simulink model "Comparative"  (R2022a)
settings: Solver=ode45  StartTime=0.0  StopTime=10  MaxStep=0.1  RelTol=1e-3  EnableMultiTasking=on
values from neighbouring files (symbols this model uses):
  fi0 = 30    [parameters.m]
  kd = 0.1537    [parameters.m]
  ki = 768.3330    (= 768.333)    [parameters.m]
  kp = 23.0500    (= 23.05)    [parameters.m]
  kp_angle = 6    [parameters.m]
  v0 = 0    [parameters.m]
libraries: fuzblock x1
settings Model: Creator=JM  LastModifiedBy=josem
settings SolverCC: AlgebraicLoopSolver=TrustRegion
settings DataIOCC: LimitDataPoints=on  SaveFormat=Array  ReturnWorkspaceOutputs=off
settings OptimizationCC: LifeSpan=inf
settings DebuggingCC: UnconnectedInputMsg=warning  UnconnectedOutputMsg=warning  UnconnectedLineMsg=warning  SFUnexpectedBacktrackingDiag=warning  SFNoUnconditionalDefaultTransitionDiag=warning  SFExecutionAtInitializationDiag=none  SFMachineParentedDataDiag=warning  ArithmeticOperatorsInVariantConditions=warning
settings HardwareCC: ProdBitPerPointer=32  ProdBitPerSizeT=32  ProdBitPerPtrDiffT=32  ProdLargestAtomicFloat=None  ProdIntDivRoundTo=Undefined  ProdEndianess=Unspecified  ProdWordSize=32  ProdHWDeviceType=32-bit Generic
settings ModelReferenceCC: PropagateSignalLabelsOutOfModel=off
settings SFSimCC: SimUseLocalCustomCode=off  CustomCodeUndefinedFunction=UseInterfaceOnly
settings RTWCC: RTWUseLocalCustomCode=off
settings CodeAppCC: StateflowObjectComments=on
settings GRTTargetCC: TargetLangStandard=C89/C90 (ANSI)
settings ConfigComp: CovMetricSettings=dw  CovSaveCumulativeToWorkspaceVar=on  CovSaveSingleToWorkspaceVar=on  CovExternalEMLEnable=off

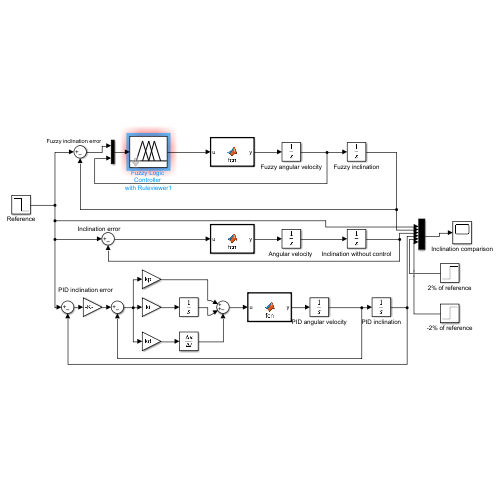
[thumbnail: Simulink's stored preview of the top-level diagram]
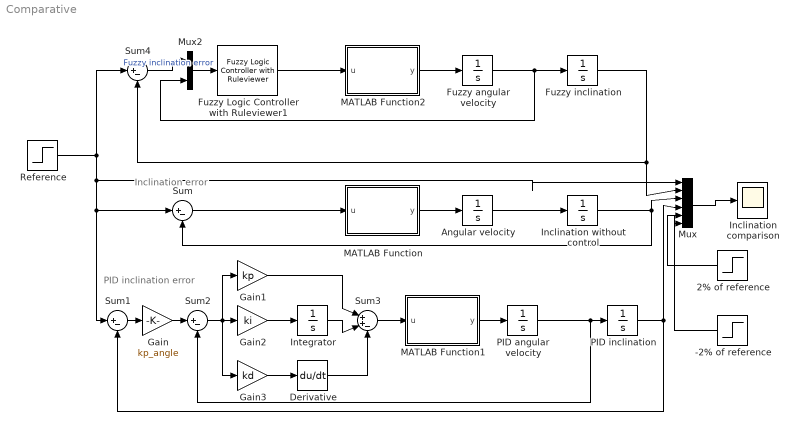
== system Comparative ==
  note: PID inclination error
  note: Inclination error
  -2% of reference : Step  Time=0  Before=-fi0*0.02  After=-fi0*0.02  SampleTime=0
  2% of reference : Step  Time=0  Before=fi0*0.02  After=fi0*0.02  SampleTime=0
  "Angular velocity " : Integrator  InitialCondition=v0
  Derivative : Derivative
  Fuzzy Logic Controller with Ruleviewer1 : fuzblock/Fuzzy Logic  Controller  with Ruleviewer  fismatrix=ControlFuzzy  Ts=0.1
  Fuzzy angular velocity : Integrator  InitialCondition=v0
  Fuzzy inclination : Integrator  InitialCondition=fi0
  Gain : Gain  Gain=kp_angle
  Gain1 : Gain  Gain=kp
  Gain2 : Gain  Gain=ki
  Gain3 : Gain  Gain=kd
  Inclination comparison : Scope
  Inclination without control : Integrator  InitialCondition=fi0
  Integrator : Integrator
  MATLAB Function : MATLAB Function  TreatAsAtomicUnit=on
  MATLAB Function1 : MATLAB Function  TreatAsAtomicUnit=on
  MATLAB Function2 : MATLAB Function  TreatAsAtomicUnit=on
  Mux : Mux  Inputs=6
  Mux2 : Mux  Inputs=2
  PID angular velocity : Integrator  InitialCondition=v0
  PID inclination : Integrator  InitialCondition=fi0
  Reference : Step  Before=fi0  After=0  SampleTime=0
  Sum{,1..2,4} (4 alike) : Sum  Inputs=|+-
  Sum3 : Sum  Inputs=|++-
  wires:
  "Angular velocity "/1 -> Inclination without control/1
  MATLAB Function/1(y) -> "Angular velocity "/1
  Inclination without control/1 -> Sum/2, Mux/3
  Mux/1 -> Inclination comparison/1
  Sum/1 -> MATLAB Function/1(u)
  MATLAB Function2/1(y) -> Fuzzy angular velocity/1
  Fuzzy Logic Controller with Ruleviewer1/1 -> MATLAB Function2/1(u)
  Sum4/1 -> Mux2/1  "Fuzzy inclination error"
  Mux2/1 -> Fuzzy Logic Controller with Ruleviewer1/1
  Fuzzy angular velocity/1 -> Mux2/2, Fuzzy inclination/1
  Fuzzy inclination/1 -> Mux/2, Sum4/2
  Reference/1 -> Mux/1, Sum1/1, Sum/1, Sum4/1
  MATLAB Function1/1(y) -> PID angular velocity/1
  PID inclination/1 -> Mux/4, Sum1/2
  Sum1/1 -> Gain/1
  Gain/1 -> Sum2/1
  Sum2/1 -> Gain1/1, Gain3/1, Gain2/1
  Sum3/1 -> MATLAB Function1/1(u)
  Gain2/1 -> Integrator/1
  Gain1/1 -> Sum3/1
  Integrator/1 -> Sum3/2
  Gain3/1 -> Derivative/1
  Derivative/1 -> Sum3/3
  PID angular velocity/1 -> Sum2/2, PID inclination/1
  2% of reference/1 -> Mux/5
  -2% of reference/1 -> Mux/6

== matlab function Comparative/MATLAB Function ==
  data: u input; y output
function y = fcn(u)
%#codegen
d = 0.02; % Distancia vertical del Flap hasta el C.G.
L = 0.5; % Diametro del UAV

Fsur = 1.483;% Fsur 
Keff = 0.9; % Keff
Inercia =0.0095;%Momento de inercia
KLineal=-1;%punto 45 grados (1 derivada)
Kacc=-Fsur * Keff  * (d + L/2)/Inercia;
y = u;

== matlab function Comparative/MATLAB Function2 ==
  data: u input; y output
function y = fcn(u)
%#codegen
d = 0.02; % Distancia vertical del Flap hasta el C.G.
L = 0.5; % Diametro del UAV

Fsur = 2.0614;% Fsur 
Keff = 0.9; % Keff
Inercia =0.0067;%Momento de inercia

KLineal=-1;%punto 45 grados (1 derivada)
Kacc=-Fsur * Keff  * (d + L/2)/Inercia;

y =u*Kacc*KLineal;

== matlab function Comparative/MATLAB Function1 ==
  data: u input; y output
function y = fcn(u)
%#codegen
d = 0.02; % Distancia vertical del Flap hasta el C.G.
L = 0.5; % Diametro del UAV

Fsur = 1.483;% Fsur 
Keff = 0.9; % Keff
Inercia =0.0095;%Momento de inercia
KLineal=-1;%punto 45 grados (1 derivada)
Kacc=-Fsur * Keff  * (d + L/2)/Inercia;
y = u;
